simulink model "Demo_DSRC_BSM_I_and_II_Message_cs"  (Simulink 7.6)
settings: Solver=ode5  SolverMode=SingleTasking  StartTime=0.0  StopTime=40  FixedStep=1/20  RelTol=1e-3
model workspace (MAT data in the model file):
  mbox_table : struct (value not decoded)
  model_closed = 0
  sim_status = 0
PreLoadFcn:
  | check_NUTS_defined;
  | 
  | assignin('base',['model_closed_' bdroot],false);
InitFcn:
  | PreScanExperimentInitFcn(bdroot)
StopFcn:
  | PreScanExperimentStopFcn(bdroot)
libraries: simulink x9, PreScanSimulinkLibrary x8, PreScanUsefulBlocks x5, simulink_extras x1
(part 1 of 3)
CloseFcn:
  | evalin('base',['clear model_closed_' bdroot]);
settings Model: Creator=PRESCAN  LastModifiedBy=buildbot
settings OptimizationCC: InitFltsAndDblsToZero=on
settings DebuggingCC: SaveWithParameterizedLinksMsg=none  SignalResolutionControl=TryResolveAllWithWarning  SolverPrmCheckMsg=none  MultiTaskDSMMsg=warning  MultiTaskCondExecSysMsg=none
settings SFSimCC: SimParseCustomCode=off
settings RTWCC: IncludeERTFirstTime=on
settings GRTTargetCC: TargetFcnLib=ansi_tfl_tmw.mat

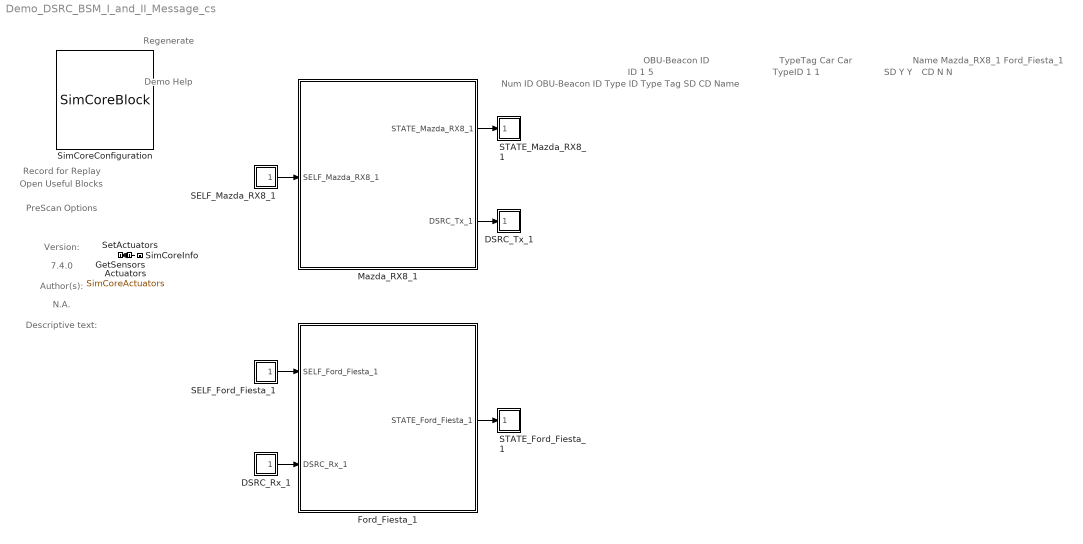
== system Demo_DSRC_BSM_I_and_II_Message_cs ==
  note: Demo Help
  note: Regenerate
  note: Record for Replay
  note: Open Useful Blocks
  note: PreScan Options
  note: Version:
  note: 7.4.0
  note: Author(s):
  note: N.A.
  note: Descriptive text:
  note: ID
      |
      | 1
      | 5
  note: OBU-Beacon ID
  note: TypeID
      |
      | 1
      | 1
  note: TypeTag
      |
      | Car
      | Car
  note: SD
      |
      | Y
      | Y
  note: CD
      |
      | N
      | N
  note: Name
      |
      | Mazda_RX8_1
      | Ford_Fiesta_1
  note: Num ID OBU-Beacon ID Type ID Type Tag SD CD Name
  Actuators : DataStoreMemory  Tag=Actuators  DataStoreName=SimCoreActuators  InitialValue=zeros(98,1)
      settings: DeleteFcn=PreScanBlockDeleteFcn;
  DSRC_Rx_1 : Subsystem  Tag=DSRC_R  Priority=3  mask(PreScan Source Block: DSRC Receiver){NrEntitiesOut=1, PortName=DSRC_Rx_1, PortIndex=16, PortWidth=91, TimeStep=1/20}
      mask prompts: NrEntitiesOut "User Specified: # of Visible Actors"; PortName "Auto Assigned: Port Name [-]"; PortIndex "Auto Assigned: Index [-]"; PortWidth "Auto Assigned: Port Dimensions [-]"; TimeStep "Auto Assigned: Upload Period [s]"
      mask help:
      | Using the DSRC Receiver (R) and Transmitter (T) information between actors can be exchanged.
      |
      | The DSRC Reciever receives actor information.
      |
      | For more information, please click Help.
      settings: DeleteFcn=PreScanBlockDeleteFcn;
      mask Help: eval('openHelp(473)')
      mask Display: image(imread('DSRCReceiver.png'))
  DSRC_Tx_1 : Subsystem  Tag=DSRC_T  Priority=0  mask(PreScan Sink Block: DSRC_T){PortName=DSRC_Tx_1, PortIndex=15, PortWidth=68, TimeStep=1/20}
      mask prompts: PortName "Auto Assigned: Port Name [-]"; PortIndex "Auto Assigned: Index [-]"; PortWidth "Auto Assigned: Port Dimensions [-]"; TimeStep "Auto Assigned: Upload Period [s]"
      mask help:
      | Using the DSRC Receiver and Transmitter information between actors can be exchanged.
      |
      | The DSRC Transmitter receives actors information.
      |
      | For more information, please click Help.
      settings: DeleteFcn=PreScanBlockDeleteFcn;
      mask Help: eval('openHelp(473)')
      mask Display: image(imread('DSRCTransmitter.png'))
  Ford_Fiesta_1 : Subsystem  Tag=WorldObjectSubSystem  InitFcn=UniqueId = '38';
      mask Display: image(imread('Ford_Fiesta.jpg'));color('white');text(0,0,' ID=5\n')
  GetSensors : Subsystem  Tag=GetSensors  Priority=2  mask(PreScan Simulation Core Block){NrOfSensors=107, TimeStep=1/20}
      mask prompts: NrOfSensors "Number of sensor values"; TimeStep "Timestep [s]"
      mask help:
      | Please do not remove this block from the PreScan compilation sheet,
      | as it contains essential configuration parameters for a PreScan simulation.
      settings: DeleteFcn=PreScanBlockDeleteFcn;
  Mazda_RX8_1 : Subsystem  Tag=WorldObjectSubSystem  InitFcn=UniqueId = '35';
      mask Display: image(imread('Mazda_RX8.jpg'));color('white');text(0,0,' ID=1\n')
  SELF_Ford_Fiesta_1 : Subsystem  Tag=SELF  Priority=3  mask(PreScan Source Block: SELF){PortName=SELF_Ford_Fiesta_1, PortIndex=8, PortWidth=8, TimeStep=1/20}
      mask prompts: PortName "Auto-Assigned: Port Name [-]"; PortIndex "Auto-Assigned: Port Index [-]"; PortWidth "Auto-Assigned: Port Dimensions"; TimeStep "Auto-Assigned: Upload Period [s]"
      mask help:
      | The SELF port shows (state) information of the actor itself. The outputs are position in the experiment's axis system and the GPS coordinates, and the object's absolute velocity and compass heading.
      |
      | For more information, please click Help.
      settings: DeleteFcn=PreScanBlockDeleteFcn;
      mask Help: eval('openHelp(462)')
      mask Display: image(imread('GPS.png'))
  SELF_Mazda_RX8_1 : Subsystem  Tag=SELF  Priority=3  mask(PreScan Source Block: SELF){PortName=SELF_Mazda_RX8_1, PortIndex=0, PortWidth=8, TimeStep=1/20}
      mask prompts: PortName "Auto-Assigned: Port Name [-]"; PortIndex "Auto-Assigned: Port Index [-]"; PortWidth "Auto-Assigned: Port Dimensions"; TimeStep "Auto-Assigned: Upload Period [s]"
      mask help:
      | The SELF port shows (state) information of the actor itself. The outputs are position in the experiment's axis system and the GPS coordinates, and the object's absolute velocity and compass heading.
      |
      | For more information, please click Help.
      settings: DeleteFcn=PreScanBlockDeleteFcn;
      mask Help: eval('openHelp(462)')
      mask Display: image(imread('GPS.png'))
  STATE_Ford_Fiesta_1 : Subsystem  Tag=State  Priority=0  mask(PreScan Sink Block: State){x0=25.344055587322369, y0=40.621716626403114, z0=0.55, Roll0=0, Pitch0=0, Yaw0=90.028121924272284, TimeStep=1/20}
      mask prompts: x0 "Ini x-position VEHICLE wrt GLOBAL axis system [m]"; y0 "Ini y-position VEHICLE wrt GLOBAL axis system [m]"; z0 "Ini z-position VEHICLE wrt GLOBAL axis system [m]"; Roll0 "Ini roll-angle BODY wrt VEHICLE axis system [deg]"; Pitch0 "Ini pitch-angle BODY wrt VEHICLE axis system [deg]"; Yaw0 "Ini yaw-angle VEHICLE wrt GLOBAL axis system [deg]"; TimeStep "Time Step [s]"
      mask help:
      | The Actor State contains a vector signal of size (9x1), containing the following signals:
      |
      | -  Position                  (x,y,z)                                     [m]
      | -  Velocity                  (vx,vy,vz)                               [m/s]
      | -  Angles                    (Roll, Pitch, Yaw)                   [rad]
      |
      | The Actor state is defined in the global axis system.
      | The state is superponed on the Initial position defined in the GUI.
      |
      | For more information, please click Help.
      settings: DeleteFcn=PreScanBlockDeleteFcn;
      mask Help: eval('openHelp(222)')
      mask Display: image(imread('State.png'))
  STATE_Mazda_RX8_1 : Subsystem  Tag=State  Priority=0  mask(PreScan Sink Block: State){x0=78.326126732768145, y0=25.413047459027823, z0=0.51, Roll0=0, Pitch0=0, Yaw0=359.2791751968474, TimeStep=1/20}
      mask prompts: x0 "Ini x-position VEHICLE wrt GLOBAL axis system [m]"; y0 "Ini y-position VEHICLE wrt GLOBAL axis system [m]"; z0 "Ini z-position VEHICLE wrt GLOBAL axis system [m]"; Roll0 "Ini roll-angle BODY wrt VEHICLE axis system [deg]"; Pitch0 "Ini pitch-angle BODY wrt VEHICLE axis system [deg]"; Yaw0 "Ini yaw-angle VEHICLE wrt GLOBAL axis system [deg]"; TimeStep "Time Step [s]"
      mask help:
      | The Actor State contains a vector signal of size (9x1), containing the following signals:
      |
      | -  Position                  (x,y,z)                                     [m]
      | -  Velocity                  (vx,vy,vz)                               [m/s]
      | -  Angles                    (Roll, Pitch, Yaw)                   [rad]
      |
      | The Actor state is defined in the global axis system.
      | The state is superponed on the Initial position defined in the GUI.
      |
      | For more information, please click Help.
      settings: DeleteFcn=PreScanBlockDeleteFcn;
      mask Help: eval('openHelp(222)')
      mask Display: image(imread('State.png'))
  SetActuators : Subsystem  Tag=SetActuators  Priority=1  mask(PreScan Simulation Core Block){TimeStep=1/20, NrOfActuators=98}
      mask prompts: TimeStep "Timestep [s]"; NrOfActuators "Number of actuator values"
      mask help:
      | Please do not remove this block from the PreScan compilation sheet,
      | as it contains essential configuration parameters for a PreScan simulation.
      settings: DeleteFcn=PreScanBlockDeleteFcn;
  SimCoreConfiguration : M-S-Function  Tag=SimCoreConfiguration  Description=00280C243E4022AF99FBDFEEE7FC50F0A130824306B32C936ADAFC7BADA046CD  FunctionName=SimCoreBlock  Parameters=ExperimentXML PortsXML SimulationCore HostName CheckStart EnableLog RfR EnableGPUAccel ShowComputationTime  mask(PreScan Simulation Core Configurator){SimulationCore=NUTS, HostName=0, CheckStart=0, prescanversion='7.4.0', EnableLog=off, RfR=0, EnableGPUAccel=off, ShowComputationTime=off}
      mask prompts: SimulationCore "Simulation Core"; HostName "Simulation Host"; CheckStart "Show START Dialog"; prescanversion "PreScan Version"; EnableLog "Create TA Log"; RfR "Record for Replay"; EnableGPUAccel "Enable GPU Acceleration"; ShowComputationTime "Show ComputationTime Scope"
      mask help:
      | Please do not remove this block from the PreScan compilation sheet,
      | as it contains essential configuration parameter for a PreScan simulation.
      mask init:
      | model = bdroot;
      | ExperimentXML = [model(1:end-3) '.pex'];
      | PortsXML = [model '_ports.pcd'];
      settings: DeleteFcn=PreScanBlockDeleteFcn;  ModelCloseFcn=assignin('base',['model_closed_' bdroot],true);
      mask Help: eval('openHelp(812)')
      mask Display: image(imread('prescanlogo.ico'))
  SimCoreInfo : Subsystem  Tag=SimCoreInfo
  wires:
  Mazda_RX8_1/1(STATE_Mazda_RX8_1) -> STATE_Mazda_RX8_1/1(State)
  SELF_Mazda_RX8_1/1(U) -> Mazda_RX8_1/1(SELF_Mazda_RX8_1)
  Mazda_RX8_1/2(DSRC_Tx_1) -> DSRC_Tx_1/1(Y)
  Ford_Fiesta_1/1(STATE_Ford_Fiesta_1) -> STATE_Ford_Fiesta_1/1(State)
  SELF_Ford_Fiesta_1/1(U) -> Ford_Fiesta_1/1(SELF_Ford_Fiesta_1)
  DSRC_Rx_1/1(U) -> Ford_Fiesta_1/2(DSRC_Rx_1)
  SetActuators/1(dummy) -> GetSensors/1(dummy)

== system Demo_DSRC_BSM_I_and_II_Message_cs/DSRC_Rx_1 ==
  Selector : Selector  IndexMode=Zero-based  IndexOptions=Starting index (dialog)  Indices=PortIndex  OutputSizes=PortWidth(1)
  U : Outport
  wires:
  [SimCoreSensors] -> Selector/1
  Selector/1 -> U/1

== system Demo_DSRC_BSM_I_and_II_Message_cs/DSRC_Tx_1 ==
  Y : Inport  SampleTime=TimeStep
  Assignment : Assignment  IndexMode=Zero-based  SampleTime=TimeStep  IndexOptions=Starting index (dialog)  Indices=PortIndex  OutputSizes=[1 1]
  Data Store Read : DataStoreRead  DataStoreName=SimCoreActuators  SampleTime=TimeStep
  Data Store Write : DataStoreWrite  DataStoreName=SimCoreActuators
  wires:
  Y/1 -> Assignment/2
  Data Store Read/1 -> Assignment/1
  Assignment/1 -> Data Store Write/1

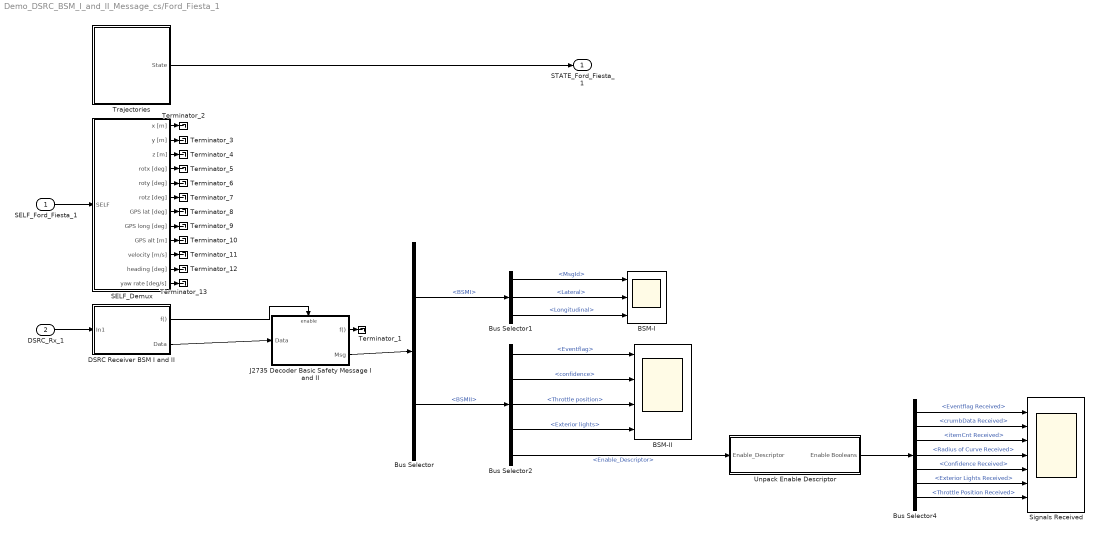
== system Demo_DSRC_BSM_I_and_II_Message_cs/Ford_Fiesta_1 ==
  SELF_Ford_Fiesta_1 : Inport  Tag=SELFInport
  DSRC_Rx_1 : Inport  Tag=DSRC_RInport  Port=2
  BSM-I : Scope  NumInputPorts=3
      settings: YMin=0~0~0  YMax=2~7500~10000
  BSM-II : Scope  NumInputPorts=4
      settings: YMin=-1~0~0~0  YMax=1~100~1~2  SaveName=ScopeData2
  Bus Selector : BusSelector  OutputSignals=BSMI,BSMII
  Bus Selector1 : BusSelector  OutputSignals=MsgId,Lateral,Longitudinal
  Bus Selector2 : BusSelector  OutputSignals=Eventflag,confidence,Throttle position,Exterior lights,Enable_Descriptor
  Bus Selector4 : BusSelector  OutputSignals=Eventflag Received,crumbData Received,itemCnt Received,Radius of Curve Received,Confidence Received,Exterior Lights Received,Throttle Position Received
  DSRC Receiver BSM I and II : Subsystem  Tag=DSRC_Receiver_BSMII
  J2735 Decoder Basic Safety Message I and II : Subsystem  Tag=J2735_Decoder_BSMII
  SELF_Demux : Subsystem  Tag=DemuxSELF
      settings: DeleteFcn=PreScanBlockDeleteFcn;
      mask Type: PreScan Demux Block:
      mask Display:
      | port_label('output',1,'x [m]')
      | port_label('output',2,'y [m]')
      | port_label('output',3,'z [m]','texmode','on')
      | port_label('output',4,'Rotx [deg]','texmode','on')
      | port_label('output',5,'Roty [deg]','texmode','on')
      | port_label('output',6,'Rotz [deg]','texmode','on')
      | port_label('output',7,'GPS lat [deg]','texmode','on')
      | port_label('output',8,'GPS long [deg]','texmode','on')
      | port_label('output',9,'GPS alt [m]','texmode','on')
      | port_label('output',10,'Velocity [m/s]')
      | port_label('output',11,'Heading [deg]')
      | port_label('output',12,'Yaw rate [deg/s]')
  Signals Received : Scope  NumInputPorts=7
      settings: YMin=-1~0~0~0~0~0~0  YMax=1~1~1~1~1~1~1  SaveName=ScopeData3
  Terminator_{1..13} (13 alike) : Terminator
  Trajectories : Subsystem  Tag=Trajectories
      settings: DeleteFcn=PreScanBlockDeleteFcn;
      mask Type: PreScan Source Block: Trajectories
      mask Description:
      | The Trajectory block contains the trajectories defined in the PreScan Experiment Editor. The output of the trajectory block is the (vehicle) State.
      | 
      | For more information, please click Help.
      mask Help: eval('openHelp(312)')
      mask Display: image(imread('Trajectory.png'));
  Unpack Enable Descriptor : Subsystem
  STATE_Ford_Fiesta_1 : Outport  Tag=StateOutport
  wires:
  Bus Selector/1 -> Bus Selector1/1  "<BSMI>"
  Bus Selector/2 -> Bus Selector2/1  "<BSMII>"
  Bus Selector2/5 -> Unpack Enable Descriptor/1(Enable_Descriptor)  "<Enable_Descriptor>"
  Bus Selector2/1 -> BSM-II/1  "<Eventflag>"
  Bus Selector1/1 -> BSM-I/1  "<MsgId>"
  Bus Selector1/2 -> BSM-I/2  "<Lateral>"
  Bus Selector1/3 -> BSM-I/3  "<Longitudinal>"
  Unpack Enable Descriptor/1(Enable Booleans) -> Bus Selector4/1
  Bus Selector4/1 -> Signals Received/1  "<Eventflag Received>"
  Bus Selector4/2 -> Signals Received/2  "<crumbData Received>"
  Bus Selector4/3 -> Signals Received/3  "<itemCnt Received>"
  Bus Selector4/4 -> Signals Received/4  "<Radius of Curve Received>"
  Bus Selector4/5 -> Signals Received/5  "<Confidence Received>"
  Bus Selector4/6 -> Signals Received/6  "<Exterior Lights Received>"
  Bus Selector4/7 -> Signals Received/7  "<Throttle Position Received>"
  Bus Selector2/3 -> BSM-II/3  "<Throttle position>"
  Bus Selector2/2 -> BSM-II/2  "<confidence>"
  Bus Selector2/4 -> BSM-II/4  "<Exterior lights>"
  SELF_Ford_Fiesta_1/1 -> SELF_Demux/1(SELF)
  DSRC Receiver BSM I and II/1(f()) -> J2735 Decoder Basic Safety Message I and II/Enable
  DSRC Receiver BSM I and II/2(Data) -> J2735 Decoder Basic Safety Message I and II/1(Data)
  DSRC_Rx_1/1 -> DSRC Receiver BSM I and II/1(In1)
  Trajectories/1(State) -> STATE_Ford_Fiesta_1/1
  J2735 Decoder Basic Safety Message I and II/2(Msg) -> Bus Selector/1
  J2735 Decoder Basic Safety Message I and II/1(f()) -> Terminator_1/1
  SELF_Demux/1(x [m]) -> Terminator_2/1
  SELF_Demux/2(y [m]) -> Terminator_3/1
  SELF_Demux/3(z [m]) -> Terminator_4/1
  SELF_Demux/4(rotx [deg]) -> Terminator_5/1
  SELF_Demux/5(roty [deg]) -> Terminator_6/1
  SELF_Demux/6(rotz [deg]) -> Terminator_7/1
  SELF_Demux/7(GPS lat [deg]) -> Terminator_8/1
  SELF_Demux/8(GPS long [deg]) -> Terminator_9/1
  SELF_Demux/9(GPS alt [m]) -> Terminator_10/1
  SELF_Demux/10(velocity [m/s]) -> Terminator_11/1
  SELF_Demux/11(heading [deg]) -> Terminator_12/1
  SELF_Demux/12(yaw rate [deg/s]) -> Terminator_13/1

== system Demo_DSRC_BSM_I_and_II_Message_cs/GetSensors ==
  dummy : Inport
  GetSensors : M-S-Function  FunctionName=GetSensorsBlock  Parameters=TimeStep NrOfSensors
  tag scope: SimCoreSensors=global
  wires:
  GetSensors/1 -> [SimCoreSensors]
  dummy/1 -> GetSensors/1

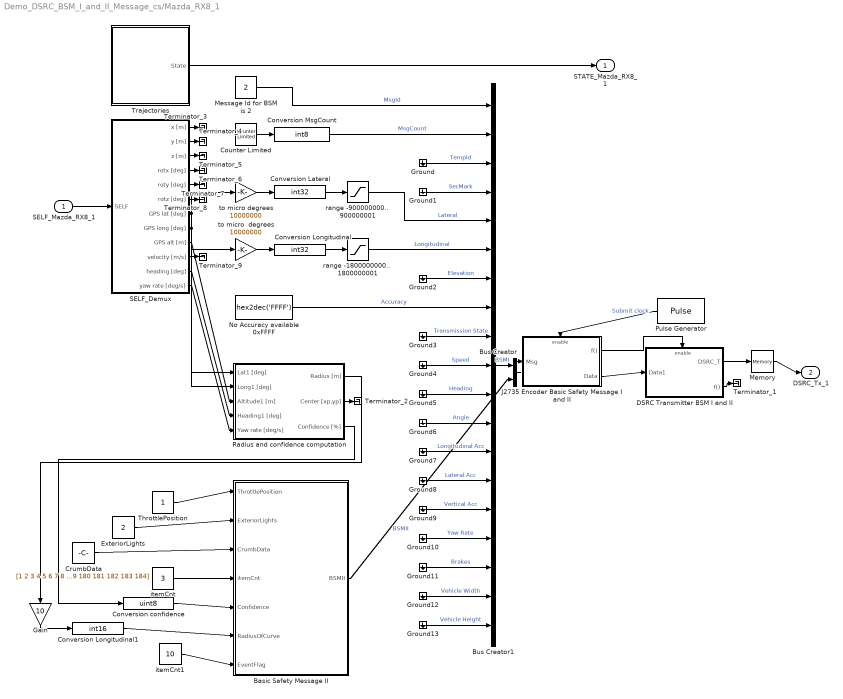
== system Demo_DSRC_BSM_I_and_II_Message_cs/Mazda_RX8_1 ==
  SELF_Mazda_RX8_1 : Inport  Tag=SELFInport
  Basic Safety Message II : Subsystem  Tag=[63 1 19 1 19 37 19 1 19 1]
      settings: CopyFcn=|
      | h=gcb;
      | val=evalin('base','DSRCT_vectenabled_Str');
      | set_param(h,'Tag',val);
      settings: PreSaveFcn=|
      | h=gcb;
      | val=get_param(h,'Tag');
      | assignin('base','DSRCT_vectenabled_Str',val);
  Bus Creator : BusCreator  Inputs=2
  Bus Creator1 : BusCreator  Inputs=19
  Conversion Lateral : DataTypeConversion  OutDataTypeStr=int32
  Conversion Longitudinal : DataTypeConversion  OutDataTypeStr=int32
  Conversion Longitudinal1 : DataTypeConversion  OutDataTypeStr=int16
  Conversion MsgCount : DataTypeConversion  OutDataTypeStr=int8
  Conversion confidence : DataTypeConversion  OutDataTypeStr=uint8
  Counter Limited : simulink/Sources/Counter Limited  SystemSampleTime=-1  uplimit=127  tsamp=-1
  CrumbData : Constant  Value=[1 2 3 4 5 6 7 8 9 10 11 12 13 14 15 16 17 18 19 20 21 22 23 24 25 26 27 28 29 30 31 32 33 34 35 36 37 38 39 40 41 42 43 44 45 46 47 48 49 50 51 52 53 54 55 56 57 58 59 60 61 62 63 64 65 66 67 68 69 70 71 72 73 74 75 76 77 78 79 80 81 82 83 84 85 86 87 88 89 90 91 92 93 94 95 96 97 98 99 100 101 102 103 104 105 106 107 108 109 110 111 112 113 114 115 116 117 118 119 120 121 122 123 124 125 126 127 128 129 130 131 132 133 134 135 136 137 138 139 140 141 142 143 144 145 146 147 148 149 150 151 152 153 154 155 156 157 158 159 160 161 162 163 164 165 166 167 168 169 170 171 172 173 174 175 176 177 178 179 180 181 182 183 184]  VectorParams1D=off  OutDataTypeStr=uint8
  DSRC Transmitter BSM I and II : Subsystem  Tag=DSRC_Transmitter_BSMII
  ExteriorLights : Constant  Value=2  OutDataTypeStr=uint8
  Gain : Gain  Gain=10
  Ground{,1..13} (14 alike) : Ground
  J2735 Encoder Basic Safety Message I and II : Subsystem  Tag=J2735_Encoder_BSMII
  Memory : Memory
  Message Id for BSM is 2 : Constant  Value=2  OutDataTypeStr=int8
  No Accuracy available 0xFFFF : Constant  Value=hex2dec('FFFF')  OutDataTypeStr=int32
  Pulse Generator : DiscretePulseGenerator  Period=1  SampleTime=1/20
  Radius and confidence computation : Subsystem  mask{GPS_origin=[0 0 0], GPS_sample_time=1/20, K_PPPATHISSTRAIGHT_M=1000}
      mask prompts: GPS_origin "GPS coordinate of the origin of the xyz coordinate system [lat lon alt]:"; GPS_sample_time "GPS coordinates sample time [s]"; K_PPPATHISSTRAIGHT_M "Radius value on a straight path (K_PPPATHISSTRAIGHT_M) [m]"
  SELF_Demux : Subsystem  Tag=DemuxSELF
      settings: DeleteFcn=PreScanBlockDeleteFcn;
      mask Type: PreScan Demux Block:
      mask Display:
      | port_label('output',1,'x [m]')
      | port_label('output',2,'y [m]')
      | port_label('output',3,'z [m]','texmode','on')
      | port_label('output',4,'Rotx [deg]','texmode','on')
      | port_label('output',5,'Roty [deg]','texmode','on')
      | port_label('output',6,'Rotz [deg]','texmode','on')
      | port_label('output',7,'GPS lat [deg]','texmode','on')
      | port_label('output',8,'GPS long [deg]','texmode','on')
      | port_label('output',9,'GPS alt [m]','texmode','on')
      | port_label('output',10,'Velocity [m/s]')
      | port_label('output',11,'Heading [deg]')
      | port_label('output',12,'Yaw rate [deg/s]')
  Terminator_{1..9} (9 alike) : Terminator
  ThrottlePosition : Constant  OutDataTypeStr=uint8
  Trajectories : Subsystem  Tag=Trajectories
      settings: DeleteFcn=PreScanBlockDeleteFcn;
      mask Type: PreScan Source Block: Trajectories
      mask Description:
      | The Trajectory block contains the trajectories defined in the PreScan Experiment Editor. The output of the trajectory block is the (vehicle) State.
      | 
      | For more information, please click Help.
      mask Help: eval('openHelp(312)')
      mask Display: image(imread('Trajectory.png'));
  itemCnt : Constant  Value=3  OutDataTypeStr=uint8
  itemCnt1 : Constant  Value=10  OutDataTypeStr=uint32
  range -1800000000..  1800000001 : Saturate  UpperLimit=1800000001  LowerLimit=-1800000000  OutDataTypeStr=int32
  range -900000000..  900000001 : Saturate  UpperLimit=900000001  LowerLimit=-900000000  OutDataTypeStr=int32
  to micro degrees : Gain  Gain=10000000
  to micro  degrees : Gain  Gain=10000000
  STATE_Mazda_RX8_1 : Outport  Tag=StateOutport
  DSRC_Tx_1 : Outport  Tag=DSRC_TOutport  Port=2
  wires:
  Message Id for BSM is 2/1 -> Bus Creator1/1  "MsgId"
  Counter Limited/1 -> Conversion MsgCount/1
  to micro  degrees/1 -> Conversion Longitudinal/1
  Conversion Longitudinal/1 -> range -1800000000..  1800000001/1
  Conversion Lateral/1 -> range -900000000..  900000001/1
  to micro degrees/1 -> Conversion Lateral/1
  No Accuracy available 0xFFFF/1 -> Bus Creator1/8  "Accuracy"
  Ground13/1 -> Bus Creator1/19  "Vehicle Height"
  Ground11/1 -> Bus Creator1/17  "Brakes"
  Ground10/1 -> Bus Creator1/16  "Yaw Rate"
  Ground9/1 -> Bus Creator1/15  "Vertical Acc"
  Ground8/1 -> Bus Creator1/14  "Lateral Acc"
  Ground7/1 -> Bus Creator1/13  "Longitudinal Acc"
  Ground6/1 -> Bus Creator1/12  "Angle"
  Ground5/1 -> Bus Creator1/11  "Heading"
  Ground4/1 -> Bus Creator1/10  "Speed"
  Ground3/1 -> Bus Creator1/9  "Transmission State"
  Ground2/1 -> Bus Creator1/7  "Elevation"
  Ground1/1 -> Bus Creator1/4  "SecMark"
  Ground/1 -> Bus Creator1/3  "TempId"
  Conversion MsgCount/1 -> Bus Creator1/2  "MsgCount"
  range -900000000..  900000001/1 -> Bus Creator1/5  "Lateral"
  range -1800000000..  1800000001/1 -> Bus Creator1/6  "Longitudinal"
  Bus Creator1/1 -> Bus Creator/1  "BSMI"
  Gain/1 -> Conversion Longitudinal1/1
  Ground12/1 -> Bus Creator1/18  "Vehicle Width"
  Radius and confidence computation/1(Radius [m]) -> Gain/1
  Radius and confidence computation/3(Confidence [%]) -> Conversion confidence/1
  SELF_Mazda_RX8_1/1 -> SELF_Demux/1(SELF)
  J2735 Encoder Basic Safety Message I and II/1(f()) -> DSRC Transmitter BSM I and II/Enable
  J2735 Encoder Basic Safety Message I and II/2(Data) -> DSRC Transmitter BSM I and II/1(Data1)
  DSRC Transmitter BSM I and II/1(DSRC_T) -> Memory/1
  Trajectories/1(State) -> STATE_Mazda_RX8_1/1
  Pulse Generator/1 -> J2735 Encoder Basic Safety Message I and II/Enable  "Submit clock"
  SELF_Demux/7(GPS lat [deg]) -> to micro degrees/1, Radius and confidence computation/1(Lat1 [deg])
  SELF_Demux/8(GPS long [deg]) -> to micro  degrees/1, Radius and confidence computation/2(Long1 [deg])
  SELF_Demux/9(GPS alt [m]) -> Radius and confidence computation/3(Altitude1 [m])
  SELF_Demux/11(heading [deg]) -> Radius and confidence computation/4(Heading1 [deg])
  SELF_Demux/12(yaw rate [deg/s]) -> Radius and confidence computation/5(Yaw rate [deg/s])
  Conversion Longitudinal1/1 -> Basic Safety Message II/6(RadiusOfCurve)
  Conversion confidence/1 -> Basic Safety Message II/5(Confidence)
  CrumbData/1 -> Basic Safety Message II/3(CrumbData)
  ExteriorLights/1 -> Basic Safety Message II/2(ExteriorLights)
  ThrottlePosition/1 -> Basic Safety Message II/1(ThrottlePosition)
  itemCnt/1 -> Basic Safety Message II/4(itemCnt)
  itemCnt1/1 -> Basic Safety Message II/7(EventFlag)
  Basic Safety Message II/1(BSMII) -> Bus Creator/2  "BSMII"
  Bus Creator/1 -> J2735 Encoder Basic Safety Message I and II/1(Msg)
  Memory/1 -> DSRC_Tx_1/1
  DSRC Transmitter BSM I and II/2(f()) -> Terminator_1/1
  Radius and confidence computation/2(Center [xp,yp]) -> Terminator_2/1
  SELF_Demux/1(x [m]) -> Terminator_3/1
  SELF_Demux/2(y [m]) -> Terminator_4/1
  SELF_Demux/3(z [m]) -> Terminator_5/1
  SELF_Demux/4(rotx [deg]) -> Terminator_6/1
  SELF_Demux/5(roty [deg]) -> Terminator_7/1
  SELF_Demux/6(rotz [deg]) -> Terminator_8/1
  SELF_Demux/10(velocity [m/s]) -> Terminator_9/1

== system Demo_DSRC_BSM_I_and_II_Message_cs/SELF_Ford_Fiesta_1 ==
  Selector : Selector  IndexMode=Zero-based  IndexOptions=Starting index (dialog)  Indices=PortIndex  OutputSizes=PortWidth(1)
  U : Outport
  wires:
  Selector/1 -> U/1
  [SimCoreSensors] -> Selector/1

== system Demo_DSRC_BSM_I_and_II_Message_cs/SELF_Mazda_RX8_1 ==
  Selector : Selector  IndexMode=Zero-based  IndexOptions=Starting index (dialog)  Indices=PortIndex  OutputSizes=PortWidth(1)
  U : Outport
  wires:
  Selector/1 -> U/1
  [SimCoreSensors] -> Selector/1

== system Demo_DSRC_BSM_I_and_II_Message_cs/STATE_Ford_Fiesta_1 ==
  State : Inport  SampleTime=TimeStep
  Acceleration : Subsystem  mask(ToSensorWorld){PortName=Acceleration_Ford_Fiesta_1, PortIndex=89, PortWidth=3, TimeStep=1/20}
      mask prompts: PortName "Port Name [-]"; PortIndex "Index [-]"; PortWidth "Port Dimensions [-]"; TimeStep "Upload Period [s]"
      mask help: Sends signal(s) from Simulink to the Sensor World
      mask Help:
      | Sends signal(s) from Simulink to the Sensor World.
      | 
      | - Port Name [-]: specifies the name of the output terminal of the Simulink block.
      | - Index [-]: specifies the start position in the output vector sent to the Sensor World
      | - Port dimensions [-]: specifies the width (number of scalars) of the output port
      | - Upload period [s]: specifies the upload period (in seconds) of the port.
      mask Display: port_label('input', 1, PortName)
  Demux : Demux  Outputs=5
  Position : Subsystem  mask(ToSensorWorld){PortName=Position_Ford_Fiesta_1, PortIndex=83, PortWidth=3, TimeStep=1/20}
      mask prompts: PortName "Port Name [-]"; PortIndex "Index [-]"; PortWidth "Port Dimensions [-]"; TimeStep "Upload Period [s]"
      mask help: Sends signal(s) from Simulink to the Sensor World
      mask Help:
      | Sends signal(s) from Simulink to the Sensor World.
      | 
      | - Port Name [-]: specifies the name of the output terminal of the Simulink block.
      | - Index [-]: specifies the start position in the output vector sent to the Sensor World
      | - Port dimensions [-]: specifies the width (number of scalars) of the output port
      | - Upload period [s]: specifies the upload period (in seconds) of the port.
      mask Display: port_label('input', 1, PortName)
  RPY : Subsystem  mask(ToSensorWorld){PortName=RPY_Ford_Fiesta_1, PortIndex=92, PortWidth=3, TimeStep=1/20}
      mask prompts: PortName "Port Name [-]"; PortIndex "Index [-]"; PortWidth "Port Dimensions [-]"; TimeStep "Upload Period [s]"
      mask help: Sends signal(s) from Simulink to the Sensor World
      mask Help:
      | Sends signal(s) from Simulink to the Sensor World.
      | 
      | - Port Name [-]: specifies the name of the output terminal of the Simulink block.
      | - Index [-]: specifies the start position in the output vector sent to the Sensor World
      | - Port dimensions [-]: specifies the width (number of scalars) of the output port
      | - Upload period [s]: specifies the upload period (in seconds) of the port.
      mask Display: port_label('input', 1, PortName)
  Velocity : Subsystem  mask(ToSensorWorld){PortName=Velocity_Ford_Fiesta_1, PortIndex=86, PortWidth=3, TimeStep=1/20}
      mask prompts: PortName "Port Name [-]"; PortIndex "Index [-]"; PortWidth "Port Dimensions [-]"; TimeStep "Upload Period [s]"
      mask help: Sends signal(s) from Simulink to the Sensor World
      mask Help:
      | Sends signal(s) from Simulink to the Sensor World.
      | 
      | - Port Name [-]: specifies the name of the output terminal of the Simulink block.
      | - Index [-]: specifies the start position in the output vector sent to the Sensor World
      | - Port dimensions [-]: specifies the width (number of scalars) of the output port
      | - Upload period [s]: specifies the upload period (in seconds) of the port.
      mask Display: port_label('input', 1, PortName)
  iniBODYAngles wrtVEH [rad] : Constant  Value=[Roll0 Pitch0 0]  SampleTime=TimeStep
  iniVEHAngles wrtGLOB [rad] : Constant  Value=[0 0 Yaw0]  SampleTime=TimeStep
  iniVEHposition wrtGLOB [m] : Constant  Value=[x0 y0 z0]  SampleTime=TimeStep
  state2FullState : PreScanSimulinkLibrary/state2FullState  SystemSampleTime=-1
  velRPY : Subsystem  mask(ToSensorWorld){PortName=velRPY_Ford_Fiesta_1, PortIndex=95, PortWidth=3, TimeStep=1/20}
      mask prompts: PortName "Port Name [-]"; PortIndex "Index [-]"; PortWidth "Port Dimensions [-]"; TimeStep "Upload Period [s]"
      mask help: Sends signal(s) from Simulink to the Sensor World
      mask Help:
      | Sends signal(s) from Simulink to the Sensor World.
      | 
      | - Port Name [-]: specifies the name of the output terminal of the Simulink block.
      | - Index [-]: specifies the start position in the output vector sent to the Sensor World
      | - Port dimensions [-]: specifies the width (number of scalars) of the output port
      | - Upload period [s]: specifies the upload period (in seconds) of the port.
      mask Display: port_label('input', 1, PortName)
  wires:
  Demux/5 -> velRPY/1(Y)
  Demux/4 -> RPY/1(Y)
  Demux/3 -> Acceleration/1(Y)
  Demux/2 -> Velocity/1(Y)
  Demux/1 -> Position/1(Y)
  State/1 -> state2FullState/1
  state2FullState/1 -> Demux/1
  iniVEHposition wrtGLOB [m]/1 -> state2FullState/2
  iniBODYAngles wrtVEH [rad]/1 -> state2FullState/3
  iniVEHAngles wrtGLOB [rad]/1 -> state2FullState/4

== system Demo_DSRC_BSM_I_and_II_Message_cs/STATE_Mazda_RX8_1 ==
  State : Inport  SampleTime=TimeStep
  Acceleration : Subsystem  mask(ToSensorWorld){PortName=Acceleration_Mazda_RX8_1, PortIndex=6, PortWidth=3, TimeStep=1/20}
      mask prompts: PortName "Port Name [-]"; PortIndex "Index [-]"; PortWidth "Port Dimensions [-]"; TimeStep "Upload Period [s]"
      mask help: Sends signal(s) from Simulink to the Sensor World
      mask Help:
      | Sends signal(s) from Simulink to the Sensor World.
      | 
      | - Port Name [-]: specifies the name of the output terminal of the Simulink block.
      | - Index [-]: specifies the start position in the output vector sent to the Sensor World
      | - Port dimensions [-]: specifies the width (number of scalars) of the output port
      | - Upload period [s]: specifies the upload period (in seconds) of the port.
      mask Display: port_label('input', 1, PortName)
  Demux : Demux  Outputs=5
  Position : Subsystem  mask(ToSensorWorld){PortName=Position_Mazda_RX8_1, PortIndex=0, PortWidth=3, TimeStep=1/20}
      mask prompts: PortName "Port Name [-]"; PortIndex "Index [-]"; PortWidth "Port Dimensions [-]"; TimeStep "Upload Period [s]"
      mask help: Sends signal(s) from Simulink to the Sensor World
      mask Help:
      | Sends signal(s) from Simulink to the Sensor World.
      | 
      | - Port Name [-]: specifies the name of the output terminal of the Simulink block.
      | - Index [-]: specifies the start position in the output vector sent to the Sensor World
      | - Port dimensions [-]: specifies the width (number of scalars) of the output port
      | - Upload period [s]: specifies the upload period (in seconds) of the port.
      mask Display: port_label('input', 1, PortName)
  RPY : Subsystem  mask(ToSensorWorld){PortName=RPY_Mazda_RX8_1, PortIndex=9, PortWidth=3, TimeStep=1/20}
      mask prompts: PortName "Port Name [-]"; PortIndex "Index [-]"; PortWidth "Port Dimensions [-]"; TimeStep "Upload Period [s]"
      mask help: Sends signal(s) from Simulink to the Sensor World
      mask Help:
      | Sends signal(s) from Simulink to the Sensor World.
      | 
      | - Port Name [-]: specifies the name of the output terminal of the Simulink block.
      | - Index [-]: specifies the start position in the output vector sent to the Sensor World
      | - Port dimensions [-]: specifies the width (number of scalars) of the output port
      | - Upload period [s]: specifies the upload period (in seconds) of the port.
      mask Display: port_label('input', 1, PortName)
  Velocity : Subsystem  mask(ToSensorWorld){PortName=Velocity_Mazda_RX8_1, PortIndex=3, PortWidth=3, TimeStep=1/20}
      mask prompts: PortName "Port Name [-]"; PortIndex "Index [-]"; PortWidth "Port Dimensions [-]"; TimeStep "Upload Period [s]"
      mask help: Sends signal(s) from Simulink to the Sensor World
      mask Help:
      | Sends signal(s) from Simulink to the Sensor World.
      | 
      | - Port Name [-]: specifies the name of the output terminal of the Simulink block.
      | - Index [-]: specifies the start position in the output vector sent to the Sensor World
      | - Port dimensions [-]: specifies the width (number of scalars) of the output port
      | - Upload period [s]: specifies the upload period (in seconds) of the port.
      mask Display: port_label('input', 1, PortName)
  iniBODYAngles wrtVEH [rad] : Constant  Value=[Roll0 Pitch0 0]  SampleTime=TimeStep
  iniVEHAngles wrtGLOB [rad] : Constant  Value=[0 0 Yaw0]  SampleTime=TimeStep
  iniVEHposition wrtGLOB [m] : Constant  Value=[x0 y0 z0]  SampleTime=TimeStep
  state2FullState : PreScanSimulinkLibrary/state2FullState  SystemSampleTime=-1
  velRPY : Subsystem  mask(ToSensorWorld){PortName=velRPY_Mazda_RX8_1, PortIndex=12, PortWidth=3, TimeStep=1/20}
      mask prompts: PortName "Port Name [-]"; PortIndex "Index [-]"; PortWidth "Port Dimensions [-]"; TimeStep "Upload Period [s]"
      mask help: Sends signal(s) from Simulink to the Sensor World
      mask Help:
      | Sends signal(s) from Simulink to the Sensor World.
      | 
      | - Port Name [-]: specifies the name of the output terminal of the Simulink block.
      | - Index [-]: specifies the start position in the output vector sent to the Sensor World
      | - Port dimensions [-]: specifies the width (number of scalars) of the output port
      | - Upload period [s]: specifies the upload period (in seconds) of the port.
      mask Display: port_label('input', 1, PortName)
  wires:
  Demux/5 -> velRPY/1(Y)
  Demux/4 -> RPY/1(Y)
  Demux/3 -> Acceleration/1(Y)
  Demux/2 -> Velocity/1(Y)
  Demux/1 -> Position/1(Y)
  State/1 -> state2FullState/1
  state2FullState/1 -> Demux/1
  iniVEHposition wrtGLOB [m]/1 -> state2FullState/2
  iniBODYAngles wrtVEH [rad]/1 -> state2FullState/3
  iniVEHAngles wrtGLOB [rad]/1 -> state2FullState/4

== system Demo_DSRC_BSM_I_and_II_Message_cs/SetActuators ==
  Bus Creator : BusCreator  Inputs=1
  Data Store Read : DataStoreRead  DataStoreName=SimCoreActuators  SampleTime=TimeStep
  SendActuators : M-S-Function  FunctionName=SendActuatorsBlock  Parameters=TimeStep NrOfActuators
  dummy : Outport
  tag scope: SimCoreInfo=global
  wires:
  Bus Creator/1 -> [SimCoreInfo]  "SimCore"
  SendActuators/2 -> Bus Creator/1  "ComputationTime[s]"
  SendActuators/1 -> dummy/1
  Data Store Read/1 -> SendActuators/1

== system Demo_DSRC_BSM_I_and_II_Message_cs/SimCoreInfo ==
  Bus Selector : BusSelector  OutputSignals=ComputationTime[s]
  Time : Scope
      settings: TimeRange=10  YMin=0  YMax=0.5  SaveName=ComputationTime
  wires:
  Bus Selector/1 -> Time/1  "<ComputationTime[s]>"
  [SimCoreInfo] -> Bus Selector/1

== system Demo_DSRC_BSM_I_and_II_Message_cs/Ford_Fiesta_1/DSRC Receiver BSM I and II ==
  In1 : Inport
  Always Enabled : Constant
  Bus Selector : BusSelector  OutputSignals=spare_1,spare_2,spare_3,spare_4,spare_5,spare_6,spare_7,spare_8,spare_9,spare_10,spare_11,spare_12,spare_13,spare_14,spare_15,spare_16,spare_17,spare_18,spare_19,spare_20,spare_21,spare_22,spare_23,spare_24,spare_25,spare_26,spare_27,spare_28,spare_29,spare_30,spare_31,spare_32,spare_33,spare_34,spare_35,spare_36,spare_37,spare_38,spare_39,spare_40,spare_41,spare_42,spare_43,spare_44,spare_45,spare_46,spare_47,spare_48,spare_49,spare_50,spare_51,spare_52,spare_53,spare_54,spare_55,spare_56,spare_57,spare_58,spare_59,spare_60,spare_61,spare_62,spare_63  OutputAsBus=on
  Bus to Vector : BusToVector
  DSRC_Rx_Demux : Subsystem  Tag=DemuxDSRCR
      settings: DeleteFcn=PreScanBlockDeleteFcn;
      mask Type: PreScan Demux Block:
      mask Display:
      | port_label('output', 1, 'Vehicle_ID')
      | port_label('output', 2, 'GPS Pos Lat [deg]')
      | port_label('output', 3, 'GPS Pos Long [deg]')
      | port_label('output', 4, 'GPS Pos Alt [m]')
      | port_label('output', 5, 'Velocity [m/s]')
      | port_label('output', 6, 'Acceleration [m/s2]')
      | port_label('output', 7, 'Heading [deg]')
      | port_label('output', 8, 'Warning signal ID')
      | port_label('output', 9, 'Maneuvre ID')
      | port_label('output', 10, 'Vehicle Type')
      | port_label('output', 11, 'Braking Capacity')
      | port_label('output', 12, 'Vehicle Size')
      | port_label('output', 13, 'Spare')
  Terminator_{1..10,12..13} (12 alike) : Terminator
  f() : Outport
  Data : Outport  Port=2
  wires:
  DSRC_Rx_Demux/1(Vehicle_ID) -> Terminator_12/1
  DSRC_Rx_Demux/2(GPS_pos_lat_[deg]) -> Terminator_13/1
  In1/1 -> DSRC_Rx_Demux/1(AntennaR)
  Always Enabled/1 -> f()/1  "Enable"
  Bus Selector/1 -> Bus to Vector/1
  Bus to Vector/1 -> Data/1
  DSRC_Rx_Demux/13(spare) -> Bus Selector/1
  DSRC_Rx_Demux/3(GPS_pos_long_[deg]) -> Terminator_1/1
  DSRC_Rx_Demux/4(GPS_pos_alt_[m]) -> Terminator_2/1
  DSRC_Rx_Demux/5(Velocity_[m/s]) -> Terminator_3/1
  DSRC_Rx_Demux/6(Acceleration_[m/s2]) -> Terminator_4/1
  DSRC_Rx_Demux/7(Heading [deg]) -> Terminator_5/1
  DSRC_Rx_Demux/8(warning_signal_id) -> Terminator_6/1
  DSRC_Rx_Demux/9(maneuvre_id) -> Terminator_7/1
  DSRC_Rx_Demux/10(vehicle_type) -> Terminator_8/1
  DSRC_Rx_Demux/11(brakingcapacity) -> Terminator_9/1
  DSRC_Rx_Demux/12(vehicle_size) -> Terminator_10/1

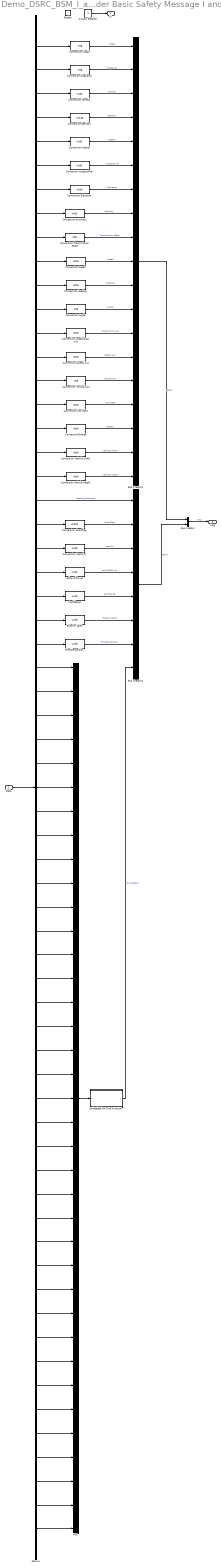
== system Demo_DSRC_BSM_I_and_II_Message_cs/Ford_Fiesta_1/J2735 Decoder Basic Safety Message I and II ==
  Data : Inport
  Enable : EnablePort  PropagateVarSize=During execution
  Always Enabled : Constant
  Bus Creator : BusCreator  Inputs=2
  Bus Creator1 : BusCreator  Inputs=19
  Bus Creator2 : BusCreator  Inputs=8
  Confidence : DataTypeConversion  OutDataTypeStr=uint8
  Conversion Accuracy : DataTypeConversion  OutDataTypeStr=int32
  Conversion Angle : DataTypeConversion  OutDataTypeStr=int8
  Conversion Brakes : DataTypeConversion  OutDataTypeStr=int16
  Conversion Elevation : DataTypeConversion  OutDataTypeStr=int16
  Conversion Heading : DataTypeConversion  OutDataTypeStr=int16
  Conversion Lateral : DataTypeConversion  OutDataTypeStr=int32
  Conversion Lateral Acc : DataTypeConversion  OutDataTypeStr=int16
  Conversion Longitudinal : DataTypeConversion  OutDataTypeStr=int32
  Conversion Longitudinal Acc : DataTypeConversion  OutDataTypeStr=int16
  Conversion MsgCount : DataTypeConversion  OutDataTypeStr=int8
  Conversion MsgId : DataTypeConversion  OutDataTypeStr=int8
  Conversion SecMark : DataTypeConversion  OutDataTypeStr=uint16
  Conversion Speed : DataTypeConversion  OutDataTypeStr=int16
  Conversion TempId : DataTypeConversion  OutDataTypeStr=int32
  Conversion Transmission State : DataTypeConversion  OutDataTypeStr=int8
  Conversion Vehicle Height : DataTypeConversion  OutDataTypeStr=int16
  Conversion Vehicle Width : DataTypeConversion  OutDataTypeStr=int16
  Conversion Vertical Acc : DataTypeConversion  OutDataTypeStr=int8
  Conversion Yaw Rate : DataTypeConversion  OutDataTypeStr=int16
  Conversion  Eventflag : DataTypeConversion  OutDataTypeStr=uint32
  Conversion  itemCnt : DataTypeConversion  OutDataTypeStr=uint8
  Demux : Demux  Outputs=63
  Embedded MATLAB Function : Stateflow chart  TreatAsAtomicUnit=on
  Exterior lights : DataTypeConversion  OutDataTypeStr=uint8
  Mux : Mux  Inputs=37
  Throttle position : DataTypeConversion  OutDataTypeStr=uint8
  radius of Curve : DataTypeConversion  OutDataTypeStr=int16
  f() : Outport  InitialOutput=[1]
  Msg : Outport  Port=2
  wires:
  Always Enabled/1 -> f()/1
  Exterior lights/1 -> Bus Creator2/6  "Exterior lights"
  Throttle position/1 -> Bus Creator2/7  "Throttle position"
  Demux/26 -> Throttle position/1
  Demux/25 -> Exterior lights/1
  Demux/24 -> Confidence/1
  Confidence/1 -> Bus Creator2/5  "confidence"
  Demux/23 -> radius of Curve/1
  radius of Curve/1 -> Bus Creator2/4  "radiusOfCurve"
  Demux/22 -> Conversion  itemCnt/1
  Conversion  itemCnt/1 -> Bus Creator2/3  "itemCnt"
  Conversion  Eventflag/1 -> Bus Creator2/2  "Eventflag"
  Demux/21 -> Conversion  Eventflag/1
  Demux/20 -> Bus Creator2/1  "Enable_Descriptor"
  Conversion Vehicle Height/1 -> Bus Creator1/19  "Vehicle Height"
  Demux/19 -> Conversion Vehicle Height/1
  Conversion Vehicle Width/1 -> Bus Creator1/18  "Vehicle Width"
  Demux/18 -> Conversion Vehicle Width/1
  Demux/17 -> Conversion Brakes/1
  Conversion Yaw Rate/1 -> Bus Creator1/16  "Yaw Rate"
  Conversion Vertical Acc/1 -> Bus Creator1/15  "Vertical Acc"
  Demux/16 -> Conversion Yaw Rate/1
  Demux/15 -> Conversion Vertical Acc/1
  Conversion Lateral Acc/1 -> Bus Creator1/14  "Lateral Acc"
  Conversion Longitudinal Acc/1 -> Bus Creator1/13  "Longitudinal Acc"
  Demux/14 -> Conversion Lateral Acc/1
  Demux/13 -> Conversion Longitudinal Acc/1
  Conversion Angle/1 -> Bus Creator1/12  "Angle"
  Conversion Heading/1 -> Bus Creator1/11  "Heading"
  Demux/12 -> Conversion Angle/1
  Demux/11 -> Conversion Heading/1
  Demux/10 -> Conversion Speed/1
  Demux/9 -> Conversion Transmission State/1
  Demux/8 -> Conversion Accuracy/1
  Conversion Elevation/1 -> Bus Creator1/7  "Elevation"
  Demux/7 -> Conversion Elevation/1
  Conversion Longitudinal/1 -> Bus Creator1/6  "Longitudinal"
  Demux/6 -> Conversion Longitudinal/1
  Conversion Lateral/1 -> Bus Creator1/5  "Lateral"
  Demux/5 -> Conversion Lateral/1
  Conversion SecMark/1 -> Bus Creator1/4  "SecMark"
  Demux/4 -> Conversion SecMark/1
  Conversion TempId/1 -> Bus Creator1/3  "TempId"
  Demux/3 -> Conversion TempId/1
  Demux/2 -> Conversion MsgCount/1
  Conversion MsgCount/1 -> Bus Creator1/2  "MsgCount"
  Conversion MsgId/1 -> Bus Creator1/1  "MsgId"
  Demux/1 -> Conversion MsgId/1
  Conversion Accuracy/1 -> Bus Creator1/8  "Accuracy"
  Conversion Transmission State/1 -> Bus Creator1/9  "Transmission State"
  Conversion Speed/1 -> Bus Creator1/10  "Speed"
  Conversion Brakes/1 -> Bus Creator1/17  "Brakes"
  Demux/27 -> Mux/1
  Demux/28 -> Mux/2
  Demux/29 -> Mux/3
  Demux/30 -> Mux/4
  Demux/31 -> Mux/5
  Demux/32 -> Mux/6
  Demux/33 -> Mux/7
  Demux/34 -> Mux/8
  Demux/35 -> Mux/9
  Demux/36 -> Mux/10
  Demux/37 -> Mux/11
  Demux/38 -> Mux/12
  Demux/39 -> Mux/13
  Demux/40 -> Mux/14
  Demux/41 -> Mux/15
  Demux/42 -> Mux/16
  Demux/43 -> Mux/17
  Demux/44 -> Mux/18
  Demux/45 -> Mux/19
  Demux/46 -> Mux/20
  Demux/47 -> Mux/21
  Demux/48 -> Mux/22
  Demux/49 -> Mux/23
  Demux/50 -> Mux/24
  Demux/51 -> Mux/25
  Demux/52 -> Mux/26
  Demux/53 -> Mux/27
  Demux/54 -> Mux/28
  Demux/55 -> Mux/29
  Demux/56 -> Mux/30
  Demux/57 -> Mux/31
  Demux/58 -> Mux/32
  Demux/59 -> Mux/33
  Demux/60 -> Mux/34
  Demux/61 -> Mux/35
  Demux/62 -> Mux/36
  Demux/63 -> Mux/37
  Mux/1 -> Embedded MATLAB Function/1(u)
  Embedded MATLAB Function/1(y) -> Bus Creator2/8  "CrumbData"
  Bus Creator2/1 -> Bus Creator/2  "BSMII"
  Bus Creator1/1 -> Bus Creator/1  "BSMI"
  Data/1 -> Demux/1
  Bus Creator/1 -> Msg/1  "Msg"

== system Demo_DSRC_BSM_I_and_II_Message_cs/Ford_Fiesta_1/SELF_Demux ==
  SELF : Inport
  Demux1 : Demux  Outputs=3
  Demux2 : Demux  Outputs=3
  Demux3 : Demux  Outputs=[3 3 1 1]
  Demux4 : Demux  Outputs=3
  Gain : Gain  Gain=180/pi
  Gain1 : Gain  Gain=180/pi
  Selector : Selector  InputPortWidth=3  IndexOptions=Index vector (dialog)  Indices=[3]  OutputSizes=1
  compas converter : Subsystem
  xyz2GPS : PreScanUsefulBlocks/xyz2GPS  CoordinateCount=1  GPS_base=[0.000000 0.000000 0.000]
  x [m] : Outport
  y [m] : Outport  Port=2
  z [m] : Outport  Port=3
  rotx [deg] : Outport  Port=4
  roty [deg] : Outport  Port=5
  rotz [deg] : Outport  Port=6
  GPS lat [deg] : Outport  Port=7
  GPS long [deg] : Outport  Port=8
  GPS alt [m] : Outport  Port=9
  velocity [m/s] : Outport  Port=10
  heading [deg] : Outport  Port=11
  yaw rate [deg/s] : Outport  Port=12
  wires:
  Demux3/4 -> Gain1/1
  Gain1/1 -> yaw rate [deg/s]/1
  Demux3/3 -> velocity [m/s]/1
  compas converter/1(heading [deg]) -> heading [deg]/1
  xyz2GPS/1 -> Demux4/1
  Demux4/3 -> GPS alt [m]/1
  Demux4/2 -> GPS long [deg]/1
  Demux4/1 -> GPS lat [deg]/1
  Demux3/2 -> Gain/1, Selector/1
  Demux3/1 -> xyz2GPS/1, Demux1/1
  SELF/1 -> Demux3/1
  Demux2/3 -> rotz [deg]/1
  Demux2/2 -> roty [deg]/1
  Demux2/1 -> rotx [deg]/1
  Demux1/3 -> z [m]/1
  Demux1/2 -> y [m]/1
  Demux1/1 -> x [m]/1
  Gain/1 -> Demux2/1
  Selector/1 -> compas converter/1(rotz [rad])

== system Demo_DSRC_BSM_I_and_II_Message_cs/Ford_Fiesta_1/Trajectories ==
  Traj2State1 : Subsystem  Tag=Traj2State
      settings: DeleteFcn=PreScanBlockDeleteFcn;
      mask Type: PreScan Demux Block:
  Trajectory_2 : Subsystem  Tag=Trajectory  mask(PreScan Source Block: Trajectory){FileName='Trajectory_2.mat', TimeStep=1/20}
      mask prompts: TimeStep "Time Step [s]"
      mask help:
      | The Trajectory block contains the trajectories defined in the PreScan Experiment Editor. The output of the trajectory block is the (vehicle) State.
      |
      | For more information, please click Help.
      mask init:
      | [direc,name]=fileparts(get_param(bdroot, 'FileName'));
      | load([direc,'/Trajectories/',FileName])
      | trajectory=trajectory';
      | 
      | traj.time=trajectory(:,1);%[];
      | traj.signals.values=trajectory(:,2:19);
      | traj.dimensions=18;
      | traj.label='';
      | 
      | SampleTime=traj.time(2)-traj.time(1);
      settings: DeleteFcn=PreScanBlockDeleteFcn;
      mask Help: eval('openHelp(312)')
      mask Display: fprintf(FileName)
  Trajectory_2_Offset : Constant  Tag=TrajectoryOffset  Value="[0  0  0  0  0  0]"
  State : Outport  Tag=TrajOutport
  wires:
  Trajectory_2/1(trajectory) -> Traj2State1/1(Traj Org)
  Trajectory_2_Offset/1 -> Traj2State1/2(Offset)
  Traj2State1/1(state) -> State/1

== system Demo_DSRC_BSM_I_and_II_Message_cs/Ford_Fiesta_1/Unpack Enable Descriptor ==
  Enable_Descriptor : Inport
  Bus Creator : BusCreator  Inputs=7
  Conversion  Confidence : DataTypeConversion  OutDataTypeStr=boolean
  Conversion  EventFlag : DataTypeConversion  OutDataTypeStr=boolean
  Conversion  ExteriorLights : DataTypeConversion  OutDataTypeStr=boolean
  Conversion  RadiusOfCurve : DataTypeConversion  OutDataTypeStr=boolean
  Conversion  ThrottlePosition : DataTypeConversion  OutDataTypeStr=boolean
  Conversion  crumbData : DataTypeConversion  OutDataTypeStr=boolean
  Conversion  itemCnt : DataTypeConversion  OutDataTypeStr=boolean
  Create enabled bitvector : Stateflow chart  TreatAsAtomicUnit=on
  Demux : Demux  Outputs=7
  Scope3 : Scope
      settings: YMin=0  YMax=130
  Enable Booleans : Outport
  wires:
  Enable_Descriptor/1 -> Create enabled bitvector/1(inp), Scope3/1
  Create enabled bitvector/1(bitvector) -> Demux/1
  Demux/1 -> Conversion  EventFlag/1  "Eventflag Received"
  Conversion  EventFlag/1 -> Bus Creator/1  "Eventflag Received"
  Demux/2 -> Conversion  crumbData/1  "crumbData Received"
  Demux/3 -> Conversion  itemCnt/1  "itemCnt Received"
  Demux/4 -> Conversion  RadiusOfCurve/1  "Radius of Curve Received"
  Demux/5 -> Conversion  Confidence/1  "Confidence Received"
  Demux/6 -> Conversion  ExteriorLights/1  "Exterior Lights Received"
  Demux/7 -> Conversion  ThrottlePosition/1  "Throttle Position Received"
  Conversion  crumbData/1 -> Bus Creator/2  "crumbData Received"
  Conversion  itemCnt/1 -> Bus Creator/3  "itemCnt Received"
  Conversion  RadiusOfCurve/1 -> Bus Creator/4  "Radius of Curve Received"
  Conversion  Confidence/1 -> Bus Creator/5  "Confidence Received"
  Conversion  ExteriorLights/1 -> Bus Creator/6  "Exterior Lights Received"
  Conversion  ThrottlePosition/1 -> Bus Creator/7  "Throttle Position Received"
  Bus Creator/1 -> Enable Booleans/1
